simulink model "wheel_speed_control"  (R2020b)
settings: Solver=VariableStepAuto  StartTime=0.0  StopTime=10.0  RelTol=1e-3  EnableMultiTasking=on
values from neighbouring files (symbols this model uses):
  d = 0.038    [init_wheel_speed_control.m]
  i_1 = 1/6.5    (= 0.153846153846)    [init_wheel_speed_control.m]
  i_2 = 1/5.6    (= 0.178571428571)    [init_wheel_speed_control.m]
  K_T = 3.45    [init_wheel_speed_control.m]
  T = 0.001    [init_wheel_speed_control.m]
settings Model: Creator=TFRICKE  LastModifiedBy=60251
settings DataIOCC: LimitDataPoints=on  ReturnWorkspaceOutputs=off
settings OptimizationCC: LifeSpan=inf
settings DebuggingCC: AllowSymbolicDim=off  SFUnexpectedBacktrackingDiag=warning  SFNoUnconditionalDefaultTransitionDiag=warning  SFExecutionAtInitializationDiag=none  ArithmeticOperatorsInVariantConditions=warning
settings ModelReferenceCC: PropagateSignalLabelsOutOfModel=off
settings SFSimCC: SimUseLocalCustomCode=off  CustomCodeUndefinedFunction=UseInterfaceOnly
settings RTWCC: RTWUseLocalCustomCode=off
settings CodeAppCC: StateflowObjectComments=on
settings GRTTargetCC: TargetLangStandard=C89/C90 (ANSI)
settings ConfigComp: CovMetricSettings=dw  CovSaveCumulativeToWorkspaceVar=on  CovSaveSingleToWorkspaceVar=on  CovExternalEMLEnable=off

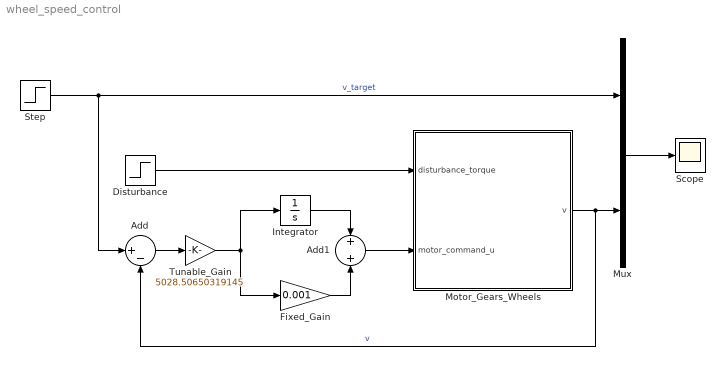
== system wheel_speed_control ==
  Add : Sum  Inputs=|+-
  Add1 : Sum
  Disturbance : Step  Time=5  After=-300  SampleTime=0
  Fixed_Gain : Gain  Gain=0.001
  Integrator : Integrator
  Motor_Gears_Wheels : Subsystem
  Mux : Mux  Inputs=2
  Scope : Scope
  Step : Step  SampleTime=0
  Tunable_Gain : Gain  Gain=5028.50650319145
  wires:
  Motor_Gears_Wheels/1(v) -> Add/2, Mux/2  "v"
  Step/1 -> Add/1, Mux/1  "v_target"
  Disturbance/1 -> Motor_Gears_Wheels/1(disturbance_torque)
  Add1/1 -> Motor_Gears_Wheels/2(motor_command_u)
  Mux/1 -> Scope/1
  Add/1 -> Tunable_Gain/1
  Tunable_Gain/1 -> Fixed_Gain/1, Integrator/1
  Integrator/1 -> Add1/1
  Fixed_Gain/1 -> Add1/2

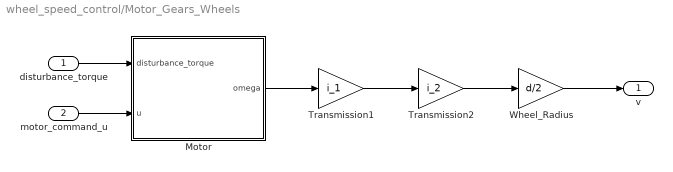
== system wheel_speed_control/Motor_Gears_Wheels ==
  disturbance_torque : Inport
  motor_command_u : Inport  Port=2
  Motor : Subsystem
  Transmission1 : Gain  Gain=i_1
  Transmission2 : Gain  Gain=i_2
  Wheel_Radius : Gain  Gain=d/2
  v : Outport  VectorParamsAs1DForOutWhenUnconnected=off
  wires:
  Transmission2/1 -> Wheel_Radius/1
  Transmission1/1 -> Transmission2/1
  Motor/1(omega) -> Transmission1/1
  motor_command_u/1 -> Motor/2(u)
  Wheel_Radius/1 -> v/1
  disturbance_torque/1 -> Motor/1(disturbance_torque)

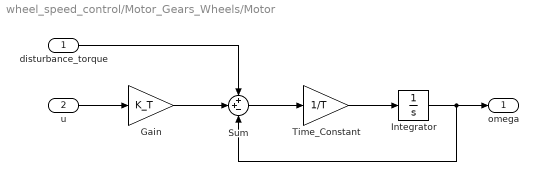
== system wheel_speed_control/Motor_Gears_Wheels/Motor ==
  disturbance_torque : Inport
  u : Inport  Port=2
  Gain : Gain  Gain=K_T
  Integrator : Integrator
  Sum : Sum  Inputs=++-
  Time_Constant : Gain  Gain=1/T
  omega : Outport  VectorParamsAs1DForOutWhenUnconnected=off
  wires:
  Gain/1 -> Sum/2
  Integrator/1 -> Sum/3, omega/1
  Sum/1 -> Time_Constant/1
  Time_Constant/1 -> Integrator/1
  u/1 -> Gain/1
  disturbance_torque/1 -> Sum/1
